simulink model "wireless"  (R2012a)
settings: Solver=ode45  StartTime=0.0  StopTime=10  RelTol=1e-3
InitFcn:
  | clear functions
undefined symbols (not defined in the file): ZigBee
libraries: truetime x5
settings Model: ExtModeAutoUpdateStatusClock=off  Creator=anton  LastModifiedBy=anton
settings DataIOCC: LimitDataPoints=on  SaveFormat=Array  SignalLoggingSaveFormat=ModelDataLogs  SaveOutput=off  SaveTime=off  ReturnWorkspaceOutputs=off
settings OptimizationCC: BlockReduction=off  BooleanDataType=off  ExpressionDepthLimit=2147483647  LifeSpan=inf  SimCompilerOptimization=Off
settings DebuggingCC: SaveWithParameterizedLinksMsg=none  UnderspecifiedInitializationDetection=Classic  MergeDetectMultiDrivingBlocksExec=none  SignalResolutionControl=TryResolveAllWithWarning  MultiTaskDSMMsg=warning  MultiTaskCondExecSysMsg=none  FcnCallInpInsideContextMsg=Use local settings  StateNameClashWarn=warning  StrictBusMsg=None  SFUnexpectedBacktrackingDiag=warning  SFNoUnconditionalDefaultTransitionDiag=warning
settings HardwareCC: ProdBitPerPointer=32  ProdLargestAtomicFloat=None  ProdIntDivRoundTo=Undefined  ProdEndianess=Unspecified  ProdWordSize=32  ProdHWDeviceType=32-bit Generic  TargetUnknown=on
settings ModelReferenceCC: PropagateSignalLabelsOutOfModel=off
settings SFSimCC: SimUseLocalCustomCode=off
settings RTWCC: RTWUseLocalCustomCode=off  RTWCompilerOptimization=Off
settings GRTTargetCC: TargetFcnLib=ansi_tfl_tmw.mat  CodeReplacementLibrary=C89/C90 (ANSI)  GeneratePreprocessorConditionals=Disable all  CombineOutputUpdateFcns=off  CPPClassGenCompliant=off  GRTInterface=on

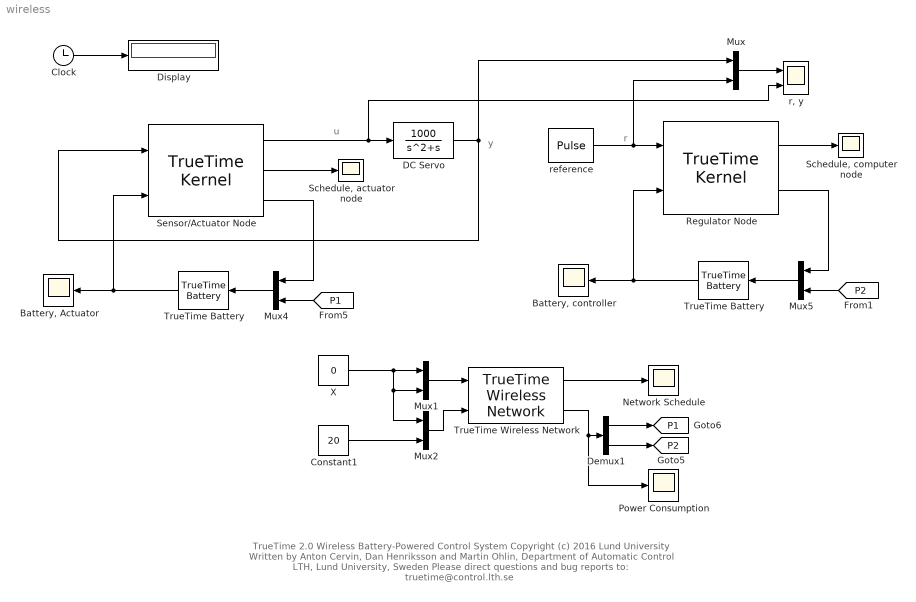
== system wireless ==
  note: u
  note: y
  note: r
  note: TrueTime 2.0  Wireless Battery-Powered Control System
      | Copyright (c) 2016 Lund University
      | Written by Anton Cervin, Dan Henriksson and Martin Ohlin,
      | Department of Automatic Control LTH, Lund University, Sweden
      | Please direct questions and bug reports to: truetime@control.lth.se
  " TrueTime Battery" : truetime/TrueTime Battery  energy=0.3
  "Battery, Actuator" : Scope
      settings: TimeRange=10  MaxDataPoints=5000  SaveToWorkspace=off  YMin=0.175  YMax=0.3  SampleTime=-1
  "Battery, controller" : Scope
      settings: TimeRange=10  MaxDataPoints=5000  SaveToWorkspace=off  SaveName=ScopeData2  YMin=0.05  YMax=0.3  SampleTime=-1
  Clock : Clock
  Constant1 : Constant  Value=20
  DC Servo : TransferFcn  Numerator=[1000]  Denominator=[1 1 0]
  Demux1 : Demux  Outputs=2
  Display : Display
  Mux{,1..2,4..5} (5 alike) : Mux  Inputs=2
  Network Schedule : Scope
      settings: TimeRange=10  MaxDataPoints=5000  SaveName=nschedule  YMin=1  YMax=2.5  SampleTime=-1
  Power Consumption : Scope
      settings: TimeRange=10  MaxDataPoints=5000  SaveToWorkspace=off  SaveName=ScopeData3  YMin=0  YMax=1  SampleTime=-1
  Regulator Node : truetime/TrueTime Kernel  sfun=regulator_init  args=[]  ninputsoutputs=[1 0]  ntriggers=0  trigtype=falling  nwnodenbr=2  clockoffsetdrift=[0 0]  schedoutput=on  battery=on  poweroutput=on  label=1: 2
  "Schedule, actuator node" : Scope
      settings: TimeRange=10  TickLabels=on  MaxDataPoints=5000  SaveToWorkspace=off  SaveName=ScopeData  YMin=1  YMax=6  SampleTime=-1  DataFormat=Array
  "Schedule, computer node" : Scope
      settings: TimeRange=10  MaxDataPoints=5000  SaveName=schedule  YMin=1  YMax=10  SampleTime=-1
  Sensor/Actuator Node : truetime/TrueTime Kernel  sfun=actuator_init  args=[]  ninputsoutputs=[1 1]  ntriggers=0  trigtype=falling  nwnodenbr=1  clockoffsetdrift=[0 0]  schedoutput=on  battery=on  poweroutput=on  label=1: 1
  TrueTime Battery : truetime/TrueTime Battery  energy=0.3
  TrueTime Wireless Network : truetime/TrueTime Wireless  Network  nwtype=802.15.4 (ZigBee)  nwnbr=1  nnodes=2  rate=800000  minsize=272  transpower=30  threshold=-48  use_pathloss_function=default  pathloss=3.5  acktimeout=0.00004  retrylimit=5  error_threshold=0.03  lossprob=0  seed=0  scheduleoutput=on  poweroutput=on
  X : Constant  Value=0
  "r, y" : Scope  NumInputPorts=2
      settings: TimeRange=10  MaxDataPoints=5000  SaveToWorkspace=off  SaveName=y  YMin=-0.717285~-5  YMax=1.85596~5  SampleTime=-1
  reference : DiscretePulseGenerator  PulseType=Time based  Period=1.2  PulseWidth=50
  tag scope: P1=global, P2=global
  wires:
  Clock/1 -> Display/1
  Mux/1 -> "r, y"/1
  DC Servo/1 -> Mux/1, Sensor/Actuator Node/1
  TrueTime Wireless Network/2 -> Demux1/1, Power Consumption/1
  Demux1/1 -> [P1]
  Demux1/2 -> [P2]
  X/1 -> Mux1/1, Mux1/2, Mux2/1
  Constant1/1 -> Mux2/2
  Mux1/1 -> TrueTime Wireless Network/1
  Mux2/1 -> TrueTime Wireless Network/2
  TrueTime Wireless Network/1 -> Network Schedule/1
  Sensor/Actuator Node/2 -> "Schedule, actuator node"/1
  Mux4/1 -> " TrueTime Battery"/1
  Sensor/Actuator Node/3 -> Mux4/1
  [P1] -> Mux4/2
  Sensor/Actuator Node/1 -> DC Servo/1, "r, y"/2
  TrueTime Battery/1 -> Regulator Node/2, "Battery, controller"/1
  Mux5/1 -> TrueTime Battery/1
  Regulator Node/2 -> Mux5/1
  [P2] -> Mux5/2
  Regulator Node/1 -> "Schedule, computer node"/1
  reference/1 -> Regulator Node/1, Mux/2
  " TrueTime Battery"/1 -> "Battery, Actuator"/1, Sensor/Actuator Node/2
